simulink model "osek_mrate"  (Simulink 6.0)
settings: Solver=FixedStepDiscrete  StartTime=0.0  StopTime=100.0  RelTol=1e-3
undefined symbols (not defined in the file or in its folder): DiscIntNeverNeededParam
libraries: simulink x4
settings Model: Creator=jcarrick  LastModifiedBy=jcarrick  ProdHWDeviceType=Motorola PowerPC
settings SolverCC: PositivePriorityOrder=on
settings DataIOCC: SaveOutput=off  SaveTime=off  SignalLoggingName=sigsOut
settings OptimizationCC: InlineInvariantSignals=off  OptimizeModelRefInitCode=on  LifeSpan=1
settings DebuggingCC: CheckExecutionContextPreStartOutputMsg=on  CheckExecutionContextRuntimeOutputMsg=on  SolverPrmCheckMsg=none
settings HardwareCC: ProdEndianess=BigEndian  ProdHWDeviceType=Motorola PowerPC
settings RTWCC: SystemTargetFile=osekworks.tlc  GenCodeOnly=on  TemplateMakefile=osek_default_tmf  GenerateReport=on  ProcessScript=osekworks_make_rtw_hook  IncludeHyperlinkInReport=on  LaunchReport=on
settings CodeAppCC: IgnoreCustomStorageClasses=off
settings STFCustomTargetCC: TargetFcnLib=ansi_tfl_tmw.mat  GenFloatMathFcnCalls=ANSI_C  ModelReferenceCompliant=off  CombineOutputUpdateFcns=on  SuppressErrorStatus=on  ERTCustomFileBanners=on  SystemTargetFile=proosek.tlc  ForcedBaseTarget=off
settings ERTTargetCC: TargetFcnLib=ansi_tfl_tmw.mat  GenFloatMathFcnCalls=ANSI_C  ModelReferenceCompliant=off  SuppressErrorStatus=on  SupportContinuousTime=on  SupportNonInlinedSFcns=on  RootIOFormat=Individual Arguments  ERTCustomFileTemplate=osek_file_process.tlc  InitialValueSource=Model
settings CustomProperty: DataType=RTWOptions_EnumType__toolbox_rtw_targets_osek_osek_osekworks_bspName  Value=phycore555
settings EnumStrPairs: String=axiomcmd565
settings SFSimCC: SFSimApplyToAllLibs=on  SFSimBuildMode=Incremental

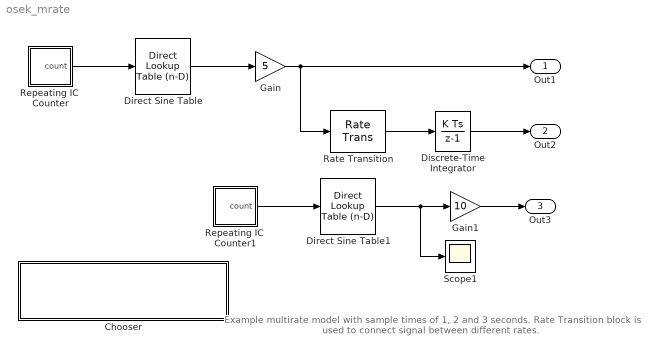
== system osek_mrate ==
  note: Example multirate model with sample times of 1, 2 and 3 seconds.
      | Rate Transition block is used to connect signal between different rates.
  Chooser : Subsystem  LoadFcn=|  PropExecContextAcrossSSBoundary=on  mask{stf=osekworks.tlc}
      | x = osek.prefs.load('osek');                               
      | Implementation = lower(x.Implementation);                  
      | clear x;                                                   
      | switch Implementation                                      
      |  case {'proosek','osekworks'}                              
      |   osek_choose_imp([Implementation,'.tlc']);                
      |   set_param(gcb,'MaskValueString',[Implementation,'.tlc']);
      |  otherwise                                                 
      |   error(['Unrecognized implementation: ' Implementation]); 
      | end                                                        
      | clear Implementation;
      mask prompts: stf "Implementation"
      mask help: Choose OSEK System Target File
      mask init:
      | osek_choose_imp(stf)
      mask StyleString: popup(osekworks.tlc|proosek.tlc)
      mask Display: disp(['Choose System Target File:\nCurrently set to "' strtok(get_param(gcs,'rtwsystemtargetfile')) '"'])
  Direct Sine Table : simulink/Lookup Tables/Direct Lookup Table (n-D)  maskTabDims=1  explicitNumDims=1  outDims=Element  tabIsInput=off  mxTable=sin(2*pi*[0:1023]/1024)  clipFlag=Error
  Direct Sine Table1 : simulink/Lookup Tables/Direct Lookup Table (n-D)  maskTabDims=1  explicitNumDims=1  outDims=Element  tabIsInput=off  mxTable=sin(2*pi*[0:1023]/1024)  clipFlag=Error
  Discrete-Time Integrator : DiscreteIntegrator  SampleTime=2  ICPrevOutput=DiscIntNeverNeededParam  ICPrevScaledInput=DiscIntNeverNeededParam
  Gain : Gain  Gain=5  SaturateOnIntegerOverflow=on
  Gain1 : Gain  Gain=10  SaturateOnIntegerOverflow=on
  Rate Transition : RateTransition
  Repeating IC  Counter : Subsystem  TreatAsAtomicUnit=on  PropExecContextAcrossSSBoundary=on  mask(CyclicCounter){ic=0, limit=1023, OutputDataType=int16, SampleTime=1}
      mask prompts: ic "Initial condition:"; limit "Counter limit:"; OutputDataType "Output data type:"; SampleTime "Sample time:"
      mask help: Count at specified sample rate from initial condition up to limit, then reset to initial condition and repeat.
      mask init:
      | set_param([gcb,'/specify type'],'DataType',OutputDataType);
      settings: RTWSystemCode=Inline
      mask StyleString: edit,edit,popup(double|single|int8|uint8|int16|uint16|int32|uint32|boolean),edit
  Repeating IC  Counter1 : Subsystem  TreatAsAtomicUnit=on  PropExecContextAcrossSSBoundary=on  mask(CyclicCounter){ic=0, limit=1023, OutputDataType=int16, SampleTime=3}
      mask prompts: ic "Initial condition:"; limit "Counter limit:"; OutputDataType "Output data type:"; SampleTime "Sample time:"
      mask help: Count at specified sample rate from initial condition up to limit, then reset to initial condition and repeat.
      mask init:
      | set_param([gcb,'/specify type'],'DataType',OutputDataType);
      settings: RTWSystemCode=Inline
      mask StyleString: edit,edit,popup(double|single|int8|uint8|int16|uint16|int32|uint32|boolean),edit
  Scope1 : Scope
      settings: TimeRange=5  YMin=-40000  YMax=40000
  Out1 : Outport
  Out2 : Outport  Port=2
  Out3 : Outport  Port=3
  wires:
  Direct Sine Table/1 -> Gain/1
  Direct Sine Table1/1 -> Gain1/1, Scope1/1
  Gain/1 -> Rate Transition/1, Out1/1
  Rate Transition/1 -> Discrete-Time Integrator/1
  Discrete-Time Integrator/1 -> Out2/1
  Gain1/1 -> Out3/1
  Repeating IC  Counter/1(count) -> Direct Sine Table/1
  Repeating IC  Counter1/1(count) -> Direct Sine Table1/1

== system osek_mrate/Chooser ==

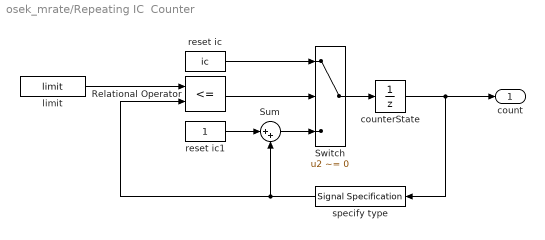
== system osek_mrate/Repeating IC  Counter ==
  Relational Operator : RelationalOperator  Operator=<=  InputSameDT=on
  Sum : Sum  Inputs=|++  InputSameDT=on
  Switch : Switch  Criteria=u2 ~= 0  Threshold=0.5  ZeroCross=off  InputSameDT=on
  counterState : UnitDelay  X0=ic  SampleTime=SampleTime
      settings: AttributesFormatString=i.c. = %<X0>
  limit : Constant  Value=limit
  reset ic : Constant  Value=ic
  reset ic1 : Constant
  specify type : simulink/Signal Attributes/Signal Specification  Orientation=left  D=-1  Ts=-1  DataType=int16  OutDataType=sfix(16)  OutScaling=2^0
      settings: SignalType=auto  SamplingMode=auto
  count : Outport
  wires:
  specify type/1 -> Relational Operator/2, Sum/2
  Relational Operator/1 -> Switch/2
  limit/1 -> Relational Operator/1
  reset ic1/1 -> Sum/1
  counterState/1 -> specify type/1, count/1
  reset ic/1 -> Switch/1
  Switch/1 -> counterState/1
  Sum/1 -> Switch/3

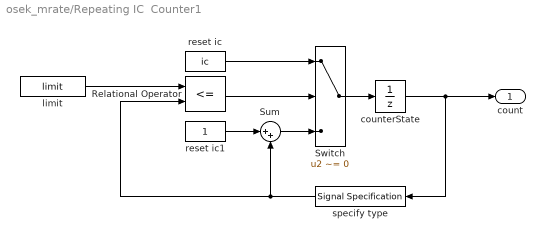
== system osek_mrate/Repeating IC  Counter1 ==
  Relational Operator : RelationalOperator  Operator=<=  InputSameDT=on
  Sum : Sum  Inputs=|++  InputSameDT=on
  Switch : Switch  Criteria=u2 ~= 0  Threshold=0.5  ZeroCross=off  InputSameDT=on
  counterState : UnitDelay  X0=ic  SampleTime=SampleTime
      settings: AttributesFormatString=i.c. = %<X0>
  limit : Constant  Value=limit
  reset ic : Constant  Value=ic
  reset ic1 : Constant
  specify type : simulink/Signal Attributes/Signal Specification  Orientation=left  D=-1  Ts=-1  DataType=int16  OutDataType=sfix(16)  OutScaling=2^0
      settings: SignalType=auto  SamplingMode=auto
  count : Outport
  wires:
  Sum/1 -> Switch/3
  Switch/1 -> counterState/1
  reset ic/1 -> Switch/1
  counterState/1 -> count/1, specify type/1
  reset ic1/1 -> Sum/1
  limit/1 -> Relational Operator/1
  Relational Operator/1 -> Switch/2
  specify type/1 -> Sum/2, Relational Operator/2
